simulink model "View_Speed"  (R2024b)
settings: Solver=FixedStepDiscrete  StartTime=0.0  StopTime=10.0  FixedStep=0.1  RelTol=1e-3  EnableMultiTasking=on
values from neighbouring files (symbols this model uses):
  C_BLANK = mpt.Parameter    [View_Speed_dd.m]
  C_CANADA = mpt.Parameter    [View_Speed_dd.m]
  C_DEFAULT_TOLER_A_VALUE = mpt.Parameter    [View_Speed_dd.m]
  C_DEFAULT_TOLER_B_VALUE = mpt.Parameter    [View_Speed_dd.m]
  C_MET_SPD_MAX_VALUE = mpt.Parameter    [View_Speed_dd.m]
  C_MET_SPD_MIN_THRESHOLD = mpt.Parameter    [View_Speed_dd.m]
  C_MEXICO = mpt.Parameter    [View_Speed_dd.m]
  C_SPEED_1KMPH = mpt.Parameter    [View_Speed_dd.m]
  C_SPEED_2KMPH = mpt.Parameter    [View_Speed_dd.m]
  C_SPEED_ZERO = mpt.Parameter    [View_Speed_dd.m]
  C_USA = mpt.Parameter    [View_Speed_dd.m]
  cFACTOR = mpt.Parameter    [View_Speed_dd.m]
  cOFFSET = mpt.Parameter    [View_Speed_dd.m]
  eTOLER_AOut = mpt.Parameter    [View_Speed_dd.m]
  eTOLER_BOut = mpt.Parameter    [View_Speed_dd.m]
  IGN_TRAN_TIMER_MS = mpt.Parameter    [View_Speed_dd.m]
  RESOLUTION_100 = mpt.Parameter    [View_Speed_dd.m]
  RTE_E_MAX_AGE_EXCEEDED = mpt.Parameter    [View_Speed_rte_types.m]
  RTE_E_NEVER_RECEIVED = mpt.Parameter    [View_Speed_rte_types.m]
  VAL_ONE = mpt.Parameter    [View_Speed_dd.m]
  View_Speed_cTaskPeriod = mpt.Parameter    [View_Speed_rte_types.m]
undefined symbols (not defined in the file or in its folder): Arr_u8_100_type_instance, Arr_u8_1024_type_instance, Arr_u8_10_type_instance, Arr_u8_128_type_instance, Arr_u8_16_type_instance, Arr_u8_17_type_instance, Arr_u8_2048_type_instance, Arr_u8_256_type_instance, Arr_u8_32_type_instance, Arr_u8_3_type_instance, Arr_u8_46_type_instance, Arr_u8_48_type_instance, Arr_u8_61_type_instance, Arr_u8_64_type_instance, Arr_u8_8_type_instance, Arr_u8_9_type_instance, CLUSTER_INACTIVE, eMET_SPDOut, eSP_ADR, eSP_CANADA, eSP_ECE, eSP_EUROPE, eSP_KOREA_FMVSS, eSP_KOREA_UN_R, eSP_MEXICO_FMVSS, eSP_MEXICO_UN_R, eSP_UK, eSP_USA, eVehicleSpeedABSIn, IgnOff, IgnOn, pJustRcvdStatus, RxCan_SignalClearJustRcvdStatus, RxCan_SignalGetJustRcvdStatus, RxCan_SignalInvalidProcessingControl, RxCan_SignalMissingProcessingControl, RxCan_SignalNRProcessingControl, SignalId, Status, tRxSignalId_type_instance, tRxSignalJustRcvdStatus_type_instance, tRxSignalStatus_type_instance, tTxSigConfirmStatus_type_instance, tTxSignalId_type_instance, TxCan_ClearCanSignalTxConfirmation
libraries: simulink x8
(part 1 of 2)
settings Model: Creator=AELANGO6  LastModifiedBy=AELANGO6
settings DataIOCC: SaveOutput=off
settings OptimizationCC: DefaultParameterBehavior=Inlined  EnhancedBackFolding=on  PassReuseOutputArgsAs=Individual arguments  ZeroExternalMemoryAtStartup=off  ZeroInternalMemoryAtStartup=off  MaxStackSize=750  OptimizeBlockOrder=speed  DifferentSizesBufferReuse=on  OptimizationCustomize=off  EfficientTunableParamExpr=on
settings DebuggingCC: ParameterTunabilityLossMsg=error
settings SFSimCC: MATLABDynamicMemAlloc=off
settings RTWCC: Description=AUTOSAR  SystemTargetFile=autosar.tlc  GenCodeOnly=on  TemplateMakefile=ert_default_tmf  PortableWordSizes=on  DataTypeReplacement=CDataTypesFixedWidth
settings CodeAppCC: ForceParamTrailComments=on  IgnoreCustomStorageClasses=off  OperatorAnnotations=on  SimulinkDataObjDesc=on  SFDataObjDesc=on  InsertBlockDesc=on
settings STFCustomTargetCC: TargetLangStandard=C99 (ISO)  MultiwordLength=256  ParMdlRefBuildCompliant=on  CompOptLevelCompliant=on  IncludeMdlTerminateFcn=off  CombineOutputUpdateFcns=on  SuppressErrorStatus=on  ERTCustomFileBanners=on  SupportNonFinite=off  SupportComplex=off  SupportContinuousTime=off  SupportNonInlinedSFcns=off  RemoveResetFunc=on  ParenthesesLevel=Maximum  CastingMode=Standards  MATLABClassNameForMDSCustomization=Simulink.SoftwareTarget.ERTCustomization  AutosarCompliant=on  UseToolchainInfoCompliant=on  LookupTableObjectStructAxisOrder=2,1,3,4,...  LUTObjectStructOrderEvenSpacing=Size,Table,Breakpoints  SystemTargetFile=autosar.tlc
settings ERTTargetCC: TargetLangStandard=C99 (ISO)  ConcurrentExecutionCompliant=off  IncludeMdlTerminateFcn=off  SuppressErrorStatus=on  SupportNonFinite=off  SupportComplex=off  ParenthesesLevel=Maximum  CastingMode=Standards  ModelStepFunctionPrototypeControlCompliant=off  CPPClassGenCompliant=off  AutosarCompliant=on  LookupTableObjectStructAxisOrder=2,1,3,4,...  LUTObjectStructOrderEvenSpacing=Size,Table,Breakpoints  ERTCustomFileTemplate=example_file_process.tlc  ERTFilePackagingFormat=CompactWithDataFile  BooleanTrueId=TRUE  BooleanFalseId=FALSE

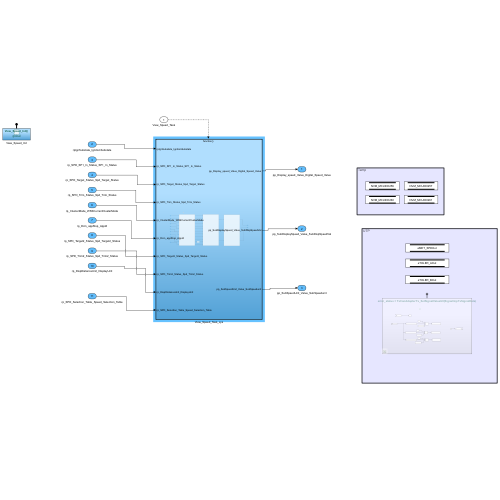
[thumbnail: Simulink's stored preview of the top-level diagram]
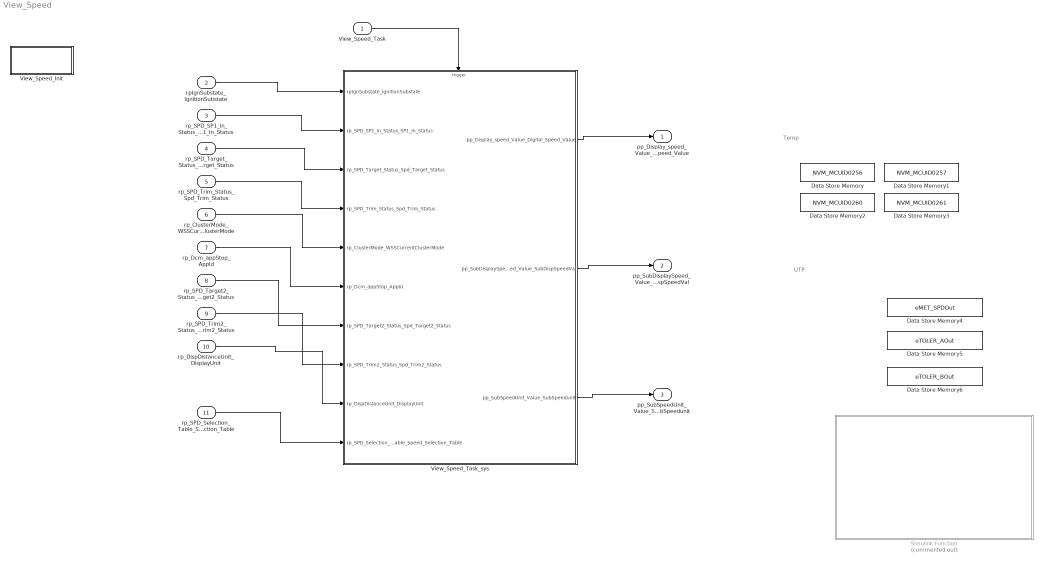
== system View_Speed ==
  note: UTP
  note: Temp
  View_Speed_Task : Inport  SampleTime=0.1  OutputFunctionCall=on
  rpIgnSubstate_IgnitionSubstate : Inport  Port=2  OutDataTypeStr=IgntionSubstateType  PortDimensions=1
  rp_SPD_SP1_In_Status_SP1_In_Status : Inport  Port=3  OutDataTypeStr=uint16  PortDimensions=1
  rp_SPD_Target_Status_Spd_Target_Status : Inport  Port=4  OutDataTypeStr=uint16  PortDimensions=1
  rp_SPD_Trim_Status_Spd_Trim_Status : Inport  Port=5  OutDataTypeStr=uint16  PortDimensions=1
  rp_ClusterMode_WSSCurrentClusterMode : Inport  Port=6  OutDataTypeStr=ClusterModes  PortDimensions=1
  rp_Dcm_appStop_AppId : Inport  Port=7  OutDataTypeStr=IOCtrl_Type  PortDimensions=1
  rp_SPD_Target2_Status_Spd_Target2_Status : Inport  Port=8  OutDataTypeStr=uint16  PortDimensions=1
  rp_SPD_Trim2_Status_Spd_Trim2_Status : Inport  Port=9  OutDataTypeStr=uint16  PortDimensions=1
  rp_DispDistanceUnit_DisplayUnit : Inport  Port=10  OutDataTypeStr=uint8  PortDimensions=1
  rp_SPD_Selection_Table_Speed_Selection_Table : Inport  Port=11  OutDataTypeStr=uint8  PortDimensions=1
  Data Store Memory : DataStoreMemory  DataStoreName=NVM_MCUID0256  ReadBeforeWriteMsg=warning  WriteAfterWriteMsg=warning  WriteAfterReadMsg=warning  InitialValue=C_MCUID0256_VALUE  ShowAdditionalParam=off  OutDataTypeStr=uint16
  Data Store Memory1 : DataStoreMemory  DataStoreName=NVM_MCUID0257  ReadBeforeWriteMsg=warning  WriteAfterWriteMsg=warning  WriteAfterReadMsg=warning  InitialValue=C_MCUID0257_VALUE  ShowAdditionalParam=off  OutDataTypeStr=uint8
  Data Store Memory2 : DataStoreMemory  DataStoreName=NVM_MCUID0260  ReadBeforeWriteMsg=warning  WriteAfterWriteMsg=warning  WriteAfterReadMsg=warning  InitialValue=C_MCUID0260_VALUE  ShowAdditionalParam=off  OutDataTypeStr=uint16
  Data Store Memory3 : DataStoreMemory  DataStoreName=NVM_MCUID0261  ReadBeforeWriteMsg=warning  WriteAfterWriteMsg=warning  WriteAfterReadMsg=warning  InitialValue=C_MCUID0261_VALUE  ShowAdditionalParam=off  OutDataTypeStr=uint8
  Data Store Memory4 : DataStoreMemory  DataStoreName=eMET_SPDOut  ReadBeforeWriteMsg=warning  WriteAfterWriteMsg=warning  WriteAfterReadMsg=warning  ShowAdditionalParam=off  OutDataTypeStr=uint16
  Data Store Memory5 : DataStoreMemory  DataStoreName=eTOLER_AOut  ReadBeforeWriteMsg=warning  WriteAfterWriteMsg=warning  WriteAfterReadMsg=warning  ShowAdditionalParam=off  OutDataTypeStr=uint16
  Data Store Memory6 : DataStoreMemory  DataStoreName=eTOLER_BOut  ReadBeforeWriteMsg=warning  WriteAfterWriteMsg=warning  WriteAfterReadMsg=warning  ShowAdditionalParam=off  OutDataTypeStr=uint16
  Simulink Function : Subsystem  Commented=on  TreatAsAtomicUnit=on
  View_Speed_Init : Subsystem  TreatAsAtomicUnit=on
  View_Speed_Task_sys : Subsystem  TreatAsAtomicUnit=on
  pp_Display_speed_Value_Digital_Speed_Value : Outport  OutDataTypeStr=uint16
  pp_SubDisplaySpeed_Value_SubDispSpeedVal : Outport  Port=2  OutDataTypeStr=uint16
  pp_SubSpeedUnit_Value_SubSpeedunit : Outport  Port=3  OutDataTypeStr=uint8
  wires:
  View_Speed_Task/1 -> View_Speed_Task_sys/Trigger
  rp_SPD_Target2_Status_Spd_Target2_Status/1 -> View_Speed_Task_sys/7(rp_SPD_Target2_Status_Spd_Target2_Status)
  rpIgnSubstate_IgnitionSubstate/1 -> View_Speed_Task_sys/1(rpIgnSubstate_IgnitionSubstate)
  rp_SPD_SP1_In_Status_SP1_In_Status/1 -> View_Speed_Task_sys/2(rp_SPD_SP1_In_Status_SP1_In_Status)
  rp_SPD_Trim_Status_Spd_Trim_Status/1 -> View_Speed_Task_sys/4(rp_SPD_Trim_Status_Spd_Trim_Status)
  rp_SPD_Target_Status_Spd_Target_Status/1 -> View_Speed_Task_sys/3(rp_SPD_Target_Status_Spd_Target_Status)
  rp_Dcm_appStop_AppId/1 -> View_Speed_Task_sys/6(rp_Dcm_appStop_AppId)
  rp_ClusterMode_WSSCurrentClusterMode/1 -> View_Speed_Task_sys/5(rp_ClusterMode_WSSCurrentClusterMode)
  rp_SPD_Trim2_Status_Spd_Trim2_Status/1 -> View_Speed_Task_sys/8(rp_SPD_Trim2_Status_Spd_Trim2_Status)
  rp_DispDistanceUnit_DisplayUnit/1 -> View_Speed_Task_sys/9(rp_DispDistanceUnit_DisplayUnit)
  View_Speed_Task_sys/2(pp_SubDisplaySpeed_Value_SubDispSpeedVal) -> pp_SubDisplaySpeed_Value_SubDispSpeedVal/1
  rp_SPD_Selection_Table_Speed_Selection_Table/1 -> View_Speed_Task_sys/10(rp_SPD_Selection_Table_Speed_Selection_Table)
  View_Speed_Task_sys/1(pp_Display_speed_Value_Digital_Speed_Value) -> pp_Display_speed_Value_Digital_Speed_Value/1
  View_Speed_Task_sys/3(pp_SubSpeedUnit_Value_SubSpeedunit) -> pp_SubSpeedUnit_Value_SubSpeedunit/1

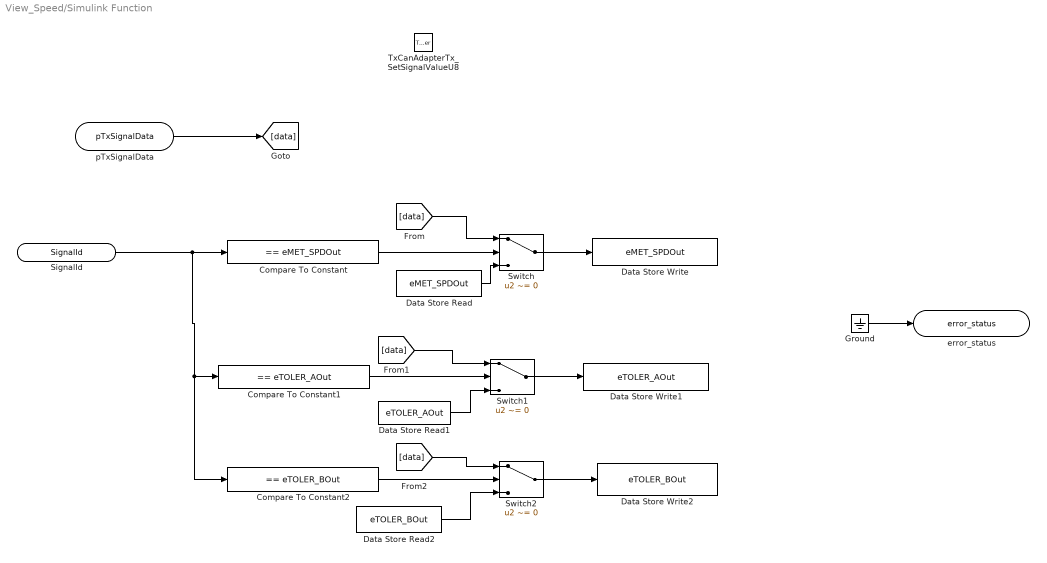
== system View_Speed/Simulink Function ==
  TxCanAdapterTx_SetSignalValueU8 : TriggerPort  TriggerType=function-call  IsSimulinkFunction=on  FunctionName=TxCanAdapterTx_SetSignalValueU8  FunctionVisibility=scoped  VariantControl=(inherit)
  Compare To Constant : simulink/Logic and Bit Operations/Compare To Constant  relop===  const=eMET_SPDOut  OutDataTypeStr=boolean
  Compare To Constant1 : simulink/Logic and Bit Operations/Compare To Constant  relop===  const=eTOLER_AOut  OutDataTypeStr=boolean
  Compare To Constant2 : simulink/Logic and Bit Operations/Compare To Constant  relop===  const=eTOLER_BOut  OutDataTypeStr=boolean
  Data Store Read : DataStoreRead  DataStoreName=eMET_SPDOut  IndexOptions=Index vector (dialog)  Indices=1  OutputSizes=1
  Data Store Read1 : DataStoreRead  DataStoreName=eTOLER_AOut  IndexOptions=Index vector (dialog)  Indices=1  OutputSizes=1
  Data Store Read2 : DataStoreRead  DataStoreName=eTOLER_BOut  IndexOptions=Index vector (dialog)  Indices=1  OutputSizes=1
  Data Store Write : DataStoreWrite  DataStoreName=eMET_SPDOut  IndexOptions=Index vector (dialog)  Indices=1  OutputSizes=1
  Data Store Write1 : DataStoreWrite  DataStoreName=eTOLER_AOut  IndexOptions=Index vector (dialog)  Indices=1  OutputSizes=1
  Data Store Write2 : DataStoreWrite  DataStoreName=eTOLER_BOut  IndexOptions=Index vector (dialog)  Indices=1  OutputSizes=1
  Ground : Ground
  Switch : Switch  Criteria=u2 ~= 0  SaturateOnIntegerOverflow=off  InputSameDT=off
  Switch1 : Switch  Criteria=u2 ~= 0  SaturateOnIntegerOverflow=off  InputSameDT=off
  Switch2 : Switch  Criteria=u2 ~= 0  SaturateOnIntegerOverflow=off  InputSameDT=off
  SignalId : ArgIn  DisableCoverage=on  OutDataTypeStr=uint16  ArgumentName=SignalId
  pTxSignalData : ArgIn  Port=2  OutDataTypeStr=uint8  ArgumentName=pTxSignalData
  error_status : ArgOut  DisableCoverage=on  OutDataTypeStr=uint8  ArgumentName=error_status
  wires:
  SignalId/1 -> Compare To Constant2/1, Compare To Constant1/1, Compare To Constant/1
  Compare To Constant/1 -> Switch/2
  Compare To Constant1/1 -> Switch1/2
  Compare To Constant2/1 -> Switch2/2
  pTxSignalData/1 -> [data]
  [data] -> Switch/1
  [data] -> Switch1/1
  [data] -> Switch2/1
  Switch/1 -> Data Store Write/1
  Switch1/1 -> Data Store Write1/1
  Switch2/1 -> Data Store Write2/1
  Data Store Read/1 -> Switch/3
  Data Store Read1/1 -> Switch1/3
  Data Store Read2/1 -> Switch2/3
  Ground/1 -> error_status/1

== system View_Speed/View_Speed_Init ==
  View_Speed_Init : TriggerPort  TriggerType=function-call  IsSimulinkFunction=on  FunctionName=View_Speed_Init  VariantControl=(inherit)

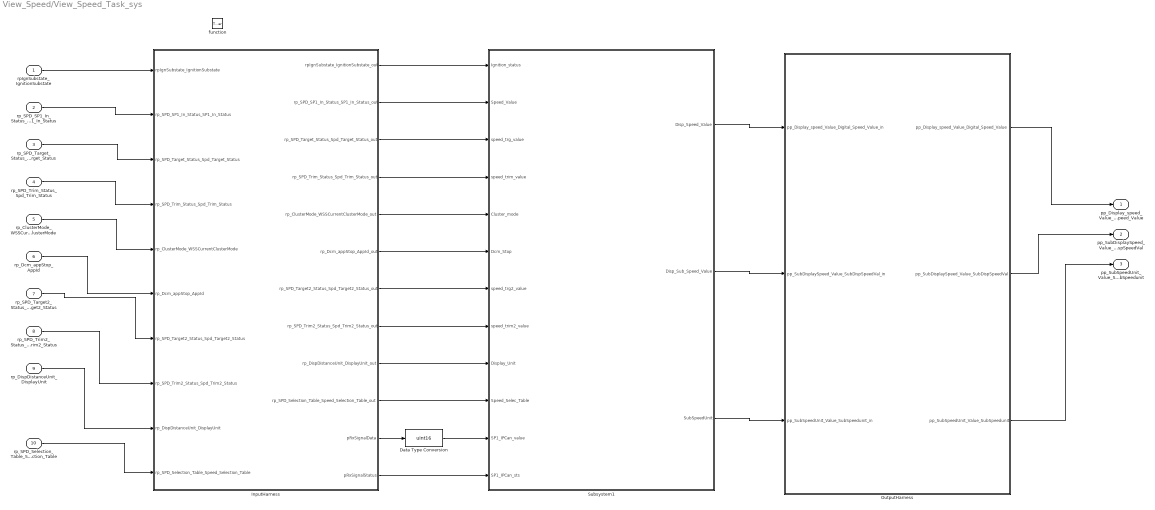
== system View_Speed/View_Speed_Task_sys ==
  rpIgnSubstate_IgnitionSubstate : Inport  OutDataTypeStr=IgntionSubstateType  PortDimensions=1
  rp_SPD_SP1_In_Status_SP1_In_Status : Inport  Port=2  OutDataTypeStr=uint16  PortDimensions=1
  rp_SPD_Target_Status_Spd_Target_Status : Inport  Port=3  OutDataTypeStr=uint16  PortDimensions=1
  rp_SPD_Trim_Status_Spd_Trim_Status : Inport  Port=4  OutDataTypeStr=uint16  PortDimensions=1
  rp_ClusterMode_WSSCurrentClusterMode : Inport  Port=5  OutDataTypeStr=ClusterModes  PortDimensions=1
  rp_Dcm_appStop_AppId : Inport  Port=6  OutDataTypeStr=IOCtrl_Type  PortDimensions=1
  rp_SPD_Target2_Status_Spd_Target2_Status : Inport  Port=7  OutDataTypeStr=uint16  PortDimensions=1
  rp_SPD_Trim2_Status_Spd_Trim2_Status : Inport  Port=8  OutDataTypeStr=uint16  PortDimensions=1
  rp_DispDistanceUnit_DisplayUnit : Inport  Port=9  OutDataTypeStr=uint8  PortDimensions=1
  rp_SPD_Selection_Table_Speed_Selection_Table : Inport  Port=10  OutDataTypeStr=uint8  PortDimensions=1
  function : TriggerPort  TriggerType=function-call  VariantControl=(inherit)  SampleTimeType=periodic  SampleTime=-1
  Data Type Conversion : DataTypeConversion  OutDataTypeStr=uint16  SaturateOnIntegerOverflow=off  RndMeth=Floor
  InputHarness : Subsystem  Variant=on
  OutputHarness : Subsystem  Variant=on
  Subsystem1 : Subsystem
  pp_Display_speed_Value_Digital_Speed_Value : Outport  OutDataTypeStr=uint16  PortDimensions=1
  pp_SubDisplaySpeed_Value_SubDispSpeedVal : Outport  Port=2  OutDataTypeStr=uint16  PortDimensions=1
  pp_SubSpeedUnit_Value_SubSpeedunit : Outport  Port=3  OutDataTypeStr=uint8  PortDimensions=1
  wires:
  rp_SPD_Trim_Status_Spd_Trim_Status/1 -> InputHarness/4(rp_SPD_Trim_Status_Spd_Trim_Status)
  rp_SPD_Target_Status_Spd_Target_Status/1 -> InputHarness/3(rp_SPD_Target_Status_Spd_Target_Status)
  rpIgnSubstate_IgnitionSubstate/1 -> InputHarness/1(rpIgnSubstate_IgnitionSubstate)
  rp_SPD_SP1_In_Status_SP1_In_Status/1 -> InputHarness/2(rp_SPD_SP1_In_Status_SP1_In_Status)
  rp_ClusterMode_WSSCurrentClusterMode/1 -> InputHarness/5(rp_ClusterMode_WSSCurrentClusterMode)
  rp_Dcm_appStop_AppId/1 -> InputHarness/6(rp_Dcm_appStop_AppId)
  rp_SPD_Target2_Status_Spd_Target2_Status/1 -> InputHarness/7(rp_SPD_Target2_Status_Spd_Target2_Status)
  rp_SPD_Trim2_Status_Spd_Trim2_Status/1 -> InputHarness/8(rp_SPD_Trim2_Status_Spd_Trim2_Status)
  rp_DispDistanceUnit_DisplayUnit/1 -> InputHarness/9(rp_DispDistanceUnit_DisplayUnit)
  rp_SPD_Selection_Table_Speed_Selection_Table/1 -> InputHarness/10(rp_SPD_Selection_Table_Speed_Selection_Table)
  OutputHarness/2(pp_SubDisplaySpeed_Value_SubDispSpeedVal) -> pp_SubDisplaySpeed_Value_SubDispSpeedVal/1
  OutputHarness/1(pp_Display_speed_Value_Digital_Speed_Value) -> pp_Display_speed_Value_Digital_Speed_Value/1
  OutputHarness/3(pp_SubSpeedUnit_Value_SubSpeedunit) -> pp_SubSpeedUnit_Value_SubSpeedunit/1
  InputHarness/1(rpIgnSubstate_IgnitionSubstate_out) -> Subsystem1/1(Ignition_status)
  InputHarness/2(rp_SPD_SP1_In_Status_SP1_In_Status_out) -> Subsystem1/2(Speed_Value)
  InputHarness/5(rp_ClusterMode_WSSCurrentClusterMode_out) -> Subsystem1/5(Cluster_mode)
  InputHarness/12(pRxSignalStatus) -> Subsystem1/12(SP1_IPCan_sts)
  InputHarness/10(rp_SPD_Selection_Table_Speed_Selection_Table_out) -> Subsystem1/10(Speed_Selec_Table)
  InputHarness/9(rp_DispDistanceUnit_DisplayUnit_out) -> Subsystem1/9(Display_Unit)
  InputHarness/8(rp_SPD_Trim2_Status_Spd_Trim2_Status_out) -> Subsystem1/8(speed_trim2_value)
  InputHarness/7(rp_SPD_Target2_Status_Spd_Target2_Status_out) -> Subsystem1/7(speed_trg2_value)
  InputHarness/6(rp_Dcm_appStop_AppId_out) -> Subsystem1/6(Dcm_Stop)
  InputHarness/4(rp_SPD_Trim_Status_Spd_Trim_Status_out) -> Subsystem1/4(speed_trim_value)
  InputHarness/3(rp_SPD_Target_Status_Spd_Target_Status_out) -> Subsystem1/3(speed_trg_value)
  Subsystem1/1(Disp_Speed_Value) -> OutputHarness/1(pp_Display_speed_Value_Digital_Speed_Value_in)
  Subsystem1/2(Disp_Sub_Speed_Value) -> OutputHarness/2(pp_SubDisplaySpeed_Value_SubDispSpeedVal_in)
  Subsystem1/3(SubSpeedUnit) -> OutputHarness/3(pp_SubSpeedUnit_Value_SubSpeedunit_in)
  InputHarness/11(pRxSignalData) -> Data Type Conversion/1
  Data Type Conversion/1 -> Subsystem1/11(SP1_IPCan_value)

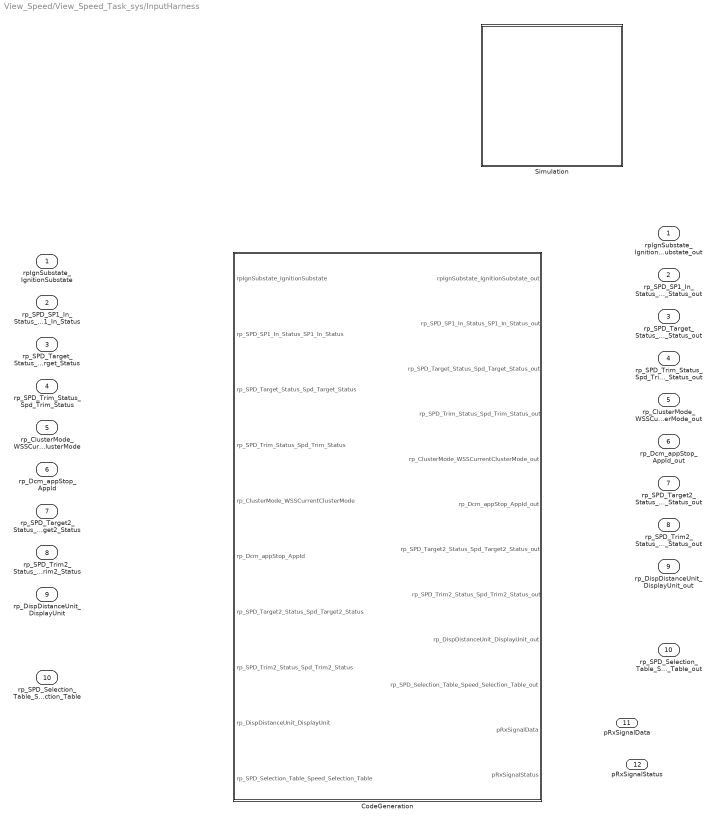
== system View_Speed/View_Speed_Task_sys/InputHarness ==
  rpIgnSubstate_IgnitionSubstate : Inport  OutDataTypeStr=IgntionSubstateType  PortDimensions=1
  rp_SPD_SP1_In_Status_SP1_In_Status : Inport  Port=2  OutDataTypeStr=uint16  PortDimensions=1
  rp_SPD_Target_Status_Spd_Target_Status : Inport  Port=3  OutDataTypeStr=uint16  PortDimensions=1
  rp_SPD_Trim_Status_Spd_Trim_Status : Inport  Port=4  OutDataTypeStr=uint16  PortDimensions=1
  rp_ClusterMode_WSSCurrentClusterMode : Inport  Port=5  OutDataTypeStr=ClusterModes  PortDimensions=1
  rp_Dcm_appStop_AppId : Inport  Port=6  OutDataTypeStr=IOCtrl_Type  PortDimensions=1
  rp_SPD_Target2_Status_Spd_Target2_Status : Inport  Port=7  OutDataTypeStr=uint16  PortDimensions=1
  rp_SPD_Trim2_Status_Spd_Trim2_Status : Inport  Port=8  OutDataTypeStr=uint16  PortDimensions=1
  rp_DispDistanceUnit_DisplayUnit : Inport  Port=9  OutDataTypeStr=uint8  PortDimensions=1
  rp_SPD_Selection_Table_Speed_Selection_Table : Inport  Port=10  OutDataTypeStr=uint8  PortDimensions=1
  CodeGeneration : Subsystem  VariantControl=CODEGENERATION
  Simulation : Subsystem  VariantControl=SIMULATION
  rpIgnSubstate_IgnitionSubstate_out : Outport  OutDataTypeStr=IgntionSubstateType  PortDimensions=1
  rp_SPD_SP1_In_Status_SP1_In_Status_out : Outport  Port=2  OutDataTypeStr=uint16  PortDimensions=1
  rp_SPD_Target_Status_Spd_Target_Status_out : Outport  Port=3  OutDataTypeStr=uint16  PortDimensions=1
  rp_SPD_Trim_Status_Spd_Trim_Status_out : Outport  Port=4  OutDataTypeStr=uint16  PortDimensions=1
  rp_ClusterMode_WSSCurrentClusterMode_out : Outport  Port=5  OutDataTypeStr=ClusterModes  PortDimensions=1
  rp_Dcm_appStop_AppId_out : Outport  Port=6  OutDataTypeStr=IOCtrl_Type  PortDimensions=1
  rp_SPD_Target2_Status_Spd_Target2_Status_out : Outport  Port=7  OutDataTypeStr=uint16  PortDimensions=1
  rp_SPD_Trim2_Status_Spd_Trim2_Status_out : Outport  Port=8  OutDataTypeStr=uint16  PortDimensions=1
  rp_DispDistanceUnit_DisplayUnit_out : Outport  Port=9  OutDataTypeStr=uint8  PortDimensions=1
  rp_SPD_Selection_Table_Speed_Selection_Table_out : Outport  Port=10  OutDataTypeStr=uint8  PortDimensions=1
  pRxSignalData : Outport  Port=11  OutDataTypeStr=uint8  VectorParamsAs1DForOutWhenUnconnected=off
  pRxSignalStatus : Outport  Port=12  OutDataTypeStr=uint8  VectorParamsAs1DForOutWhenUnconnected=off

== system View_Speed/View_Speed_Task_sys/OutputHarness ==
  pp_Display_speed_Value_Digital_Speed_Value_in : Inport  OutDataTypeStr=uint16  PortDimensions=1
  pp_SubDisplaySpeed_Value_SubDispSpeedVal_in : Inport  Port=2  OutDataTypeStr=uint16  PortDimensions=1
  pp_SubSpeedUnit_Value_SubSpeedunit_in : Inport  Port=3  OutDataTypeStr=uint8  PortDimensions=1
  CodeGeneration : Subsystem  VariantControl=CODEGENERATION
  Simulation : Subsystem  VariantControl=SIMULATION
  pp_Display_speed_Value_Digital_Speed_Value : Outport  OutDataTypeStr=uint16  PortDimensions=1
  pp_SubDisplaySpeed_Value_SubDispSpeedVal : Outport  Port=2  OutDataTypeStr=uint16  PortDimensions=1
  pp_SubSpeedUnit_Value_SubSpeedunit : Outport  Port=3  OutDataTypeStr=uint8  PortDimensions=1

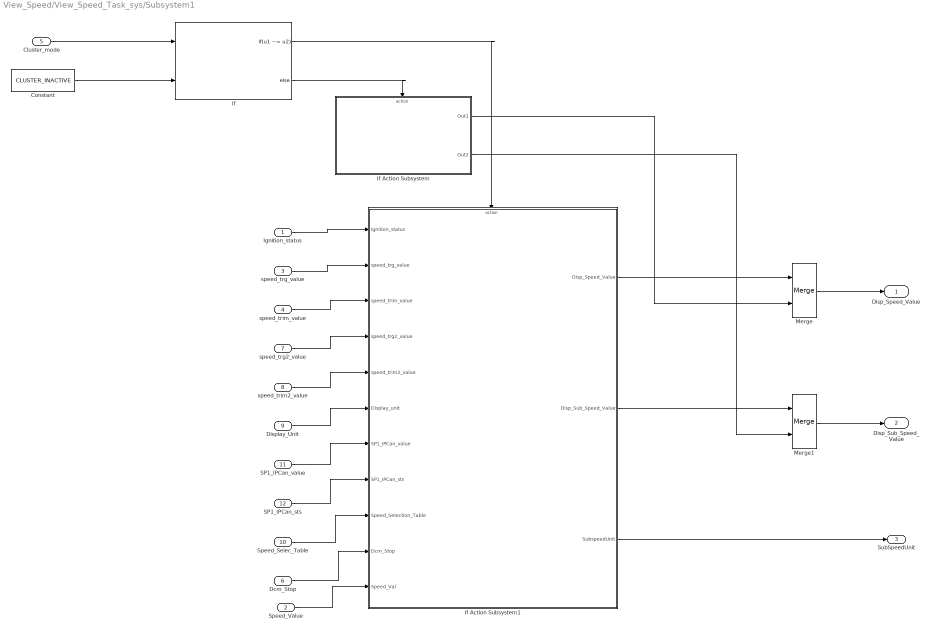
== system View_Speed/View_Speed_Task_sys/Subsystem1 ==
  Ignition_status : Inport
  Speed_Value : Inport  Port=2
  speed_trg_value : Inport  Port=3
  speed_trim_value : Inport  Port=4
  Cluster_mode : Inport  Port=5
  Dcm_Stop : Inport  Port=6
  speed_trg2_value : Inport  Port=7
  speed_trim2_value : Inport  Port=8
  Display_Unit : Inport  Port=9
  Speed_Selec_Table : Inport  Port=10  OutDataTypeStr=uint8
  SP1_IPCan_value : Inport  Port=11  OutDataTypeStr=uint16
  SP1_IPCan_sts : Inport  Port=12  OutDataTypeStr=uint8
  Constant : Constant  Value=CLUSTER_INACTIVE
  If : If  NumInputs=2  IfExpression=u1 ~= u2
  If Action Subsystem : Subsystem  TreatAsAtomicUnit=on
  If Action Subsystem1 : Subsystem  TreatAsAtomicUnit=on
  Merge : Merge
  Merge1 : Merge
  Disp_Speed_Value : Outport  VectorParamsAs1DForOutWhenUnconnected=off
  Disp_Sub_Speed_Value : Outport  Port=2  VectorParamsAs1DForOutWhenUnconnected=off
  SubSpeedUnit : Outport  Port=3  VectorParamsAs1DForOutWhenUnconnected=off
  wires:
  If/2 -> If Action Subsystem/Action
  Cluster_mode/1 -> If/1
  Constant/1 -> If/2
  If/1 -> If Action Subsystem1/Action
  Ignition_status/1 -> If Action Subsystem1/1(Ignition_status)
  speed_trg_value/1 -> If Action Subsystem1/2(speed_trg_value)
  speed_trim_value/1 -> If Action Subsystem1/3(speed_trim_value)
  Dcm_Stop/1 -> If Action Subsystem1/10(Dcm_Stop)
  speed_trim2_value/1 -> If Action Subsystem1/5(speed_trim2_value)
  speed_trg2_value/1 -> If Action Subsystem1/4(speed_trg2_value)
  SP1_IPCan_sts/1 -> If Action Subsystem1/8(SP1_IPCan_sts)
  SP1_IPCan_value/1 -> If Action Subsystem1/7(SP1_IPCan_value)
  Speed_Selec_Table/1 -> If Action Subsystem1/9(Speed_Selection_Table)
  If Action Subsystem1/1(Disp_Speed_Value) -> Merge/1
  If Action Subsystem/1(Out1) -> Merge/2
  If Action Subsystem1/2(Disp_Sub_Speed_Value) -> Merge1/1
  If Action Subsystem/2(Out2) -> Merge1/2
  Merge/1 -> Disp_Speed_Value/1
  Merge1/1 -> Disp_Sub_Speed_Value/1
  Display_Unit/1 -> If Action Subsystem1/6(Display_unit)
  If Action Subsystem1/3(SubspeedUnit) -> SubSpeedUnit/1
  Speed_Value/1 -> If Action Subsystem1/11(Speed_Val)

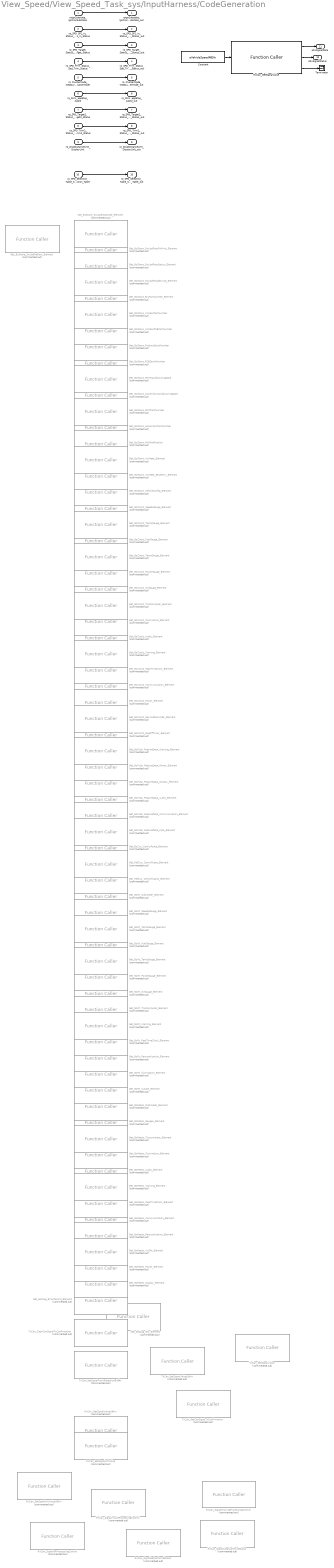
== system View_Speed/View_Speed_Task_sys/InputHarness/CodeGeneration ==
  rpIgnSubstate_IgnitionSubstate : Inport  OutDataTypeStr=IgntionSubstateType  PortDimensions=1
  rp_SPD_SP1_In_Status_SP1_In_Status : Inport  Port=2  OutDataTypeStr=uint16  PortDimensions=1
  rp_SPD_Target_Status_Spd_Target_Status : Inport  Port=3  OutDataTypeStr=uint16  PortDimensions=1
  rp_SPD_Trim_Status_Spd_Trim_Status : Inport  Port=4  OutDataTypeStr=uint16  PortDimensions=1
  rp_ClusterMode_WSSCurrentClusterMode : Inport  Port=5  OutDataTypeStr=ClusterModes  PortDimensions=1
  rp_Dcm_appStop_AppId : Inport  Port=6  OutDataTypeStr=IOCtrl_Type  PortDimensions=1
  rp_SPD_Target2_Status_Spd_Target2_Status : Inport  Port=7  OutDataTypeStr=uint16  PortDimensions=1
  rp_SPD_Trim2_Status_Spd_Trim2_Status : Inport  Port=8  OutDataTypeStr=uint16  PortDimensions=1
  rp_DispDistanceUnit_DisplayUnit : Inport  Port=9  OutDataTypeStr=uint8  PortDimensions=1
  rp_SPD_Selection_Table_Speed_Selection_Table : Inport  Port=10  OutDataTypeStr=uint8  PortDimensions=1
  Constant : Constant  Value=eVehicleSpeedABSIn
  Get_BsConst_Audio_Element : FunctionCaller  Commented=on  FunctionPrototype=[Ptr,error_status] = Get_BsConst_Audio_Element()  InputArgumentSpecifications=<Enter example>  OutputArgumentSpecifications=Arr_u8_128_type_instance(1) ,uint8(1)
  Get_BsConst_Communication_Element : FunctionCaller  Commented=on  FunctionPrototype=[Ptr,error_status] = Get_BsConst_Communication_Element()  InputArgumentSpecifications=<Enter example>  OutputArgumentSpecifications=Arr_u8_64_type_instance(1) ,uint8(1)
  Get_BsConst_EngOffTimer_Element : FunctionCaller  Commented=on  FunctionPrototype=[Ptr,error_status] = Get_BsConst_EngOffTimer_Element()  InputArgumentSpecifications=<Enter example>  OutputArgumentSpecifications=Arr_u8_32_type_instance(1) ,uint8(1)
  Get_BsConst_FuelGauge_Element : FunctionCaller  Commented=on  FunctionPrototype=[Ptr,error_status] = Get_BsConst_FuelGauge_Element()  InputArgumentSpecifications=<Enter example>  OutputArgumentSpecifications=Arr_u8_128_type_instance(1) ,uint8(1)
  Get_BsConst_Illumination_Element : FunctionCaller  Commented=on  FunctionPrototype=[Ptr,error_status] = Get_BsConst_Illumination_Element()  InputArgumentSpecifications=<Enter example>  OutputArgumentSpecifications=Arr_u8_128_type_instance(1) ,uint8(1)
  Get_BsConst_OilGauge_Element : FunctionCaller  Commented=on  FunctionPrototype=[Ptr,error_status] = Get_BsConst_OilGauge_Element()  InputArgumentSpecifications=<Enter example>  OutputArgumentSpecifications=Arr_u8_64_type_instance(1) ,uint8(1)
  Get_BsConst_PowerGauge_Element : FunctionCaller  Commented=on  FunctionPrototype=[Ptr,error_status] = Get_BsConst_PowerGauge_Element()  InputArgumentSpecifications=<Enter example>  OutputArgumentSpecifications=Arr_u8_64_type_instance(1) ,uint8(1)
  Get_BsConst_Power_Element : FunctionCaller  Commented=on  FunctionPrototype=[Ptr,error_status] = Get_BsConst_Power_Element()  InputArgumentSpecifications=<Enter example>  OutputArgumentSpecifications=Arr_u8_32_type_instance(1) ,uint8(1)
  Get_BsConst_RealTimeClock_Element : FunctionCaller  Commented=on  FunctionPrototype=[Ptr,error_status] = Get_BsConst_RealTimeClock_Element()  InputArgumentSpecifications=<Enter example>  OutputArgumentSpecifications=Arr_u8_48_type_instance(1) ,uint8(1)
  Get_BsConst_ServiceReminder_Element : FunctionCaller  Commented=on  FunctionPrototype=[Ptr,error_status] = Get_BsConst_ServiceReminder_Element()  InputArgumentSpecifications=<Enter example>  OutputArgumentSpecifications=Arr_u8_48_type_instance(1) ,uint8(1)
  Get_BsConst_SpeedoGauge_Element : FunctionCaller  Commented=on  FunctionPrototype=[Ptr,error_status] = Get_BsConst_SpeedoGauge_Element()  InputArgumentSpecifications=<Enter example>  OutputArgumentSpecifications=Arr_u8_64_type_instance(1) ,uint8(1)
  Get_BsConst_TachoGauge_Element : FunctionCaller  Commented=on  FunctionPrototype=[Ptr,error_status] = Get_BsConst_TachoGauge_Element()  InputArgumentSpecifications=<Enter example>  OutputArgumentSpecifications=Arr_u8_64_type_instance(1) ,uint8(1)
  Get_BsConst_TempGauge_Element : FunctionCaller  Commented=on  FunctionPrototype=[Ptr,error_status] = Get_BsConst_TempGauge_Element()  InputArgumentSpecifications=<Enter example>  OutputArgumentSpecifications=Arr_u8_64_type_instance(1) ,uint8(1)
  Get_BsConst_TripComputer_Element : FunctionCaller  Commented=on  FunctionPrototype=[Ptr,error_status] = Get_BsConst_TripComputer_Element()  InputArgumentSpecifications=<Enter example>  OutputArgumentSpecifications=Arr_u8_64_type_instance(1) ,uint8(1)
  Get_BsConst_Warning_Element : FunctionCaller  Commented=on  FunctionPrototype=[Ptr,error_status] = Get_BsConst_Warning_Element()  InputArgumentSpecifications=<Enter example>  OutputArgumentSpecifications=Arr_u8_64_type_instance(1) ,uint8(1)
  Get_BsCys_Certicificate_Element : FunctionCaller  Commented=on  FunctionPrototype=[Ptr,error_status] = Get_BsCys_Certicificate_Element()  InputArgumentSpecifications=<Enter example>  OutputArgumentSpecifications=Arr_u8_64_type_instance(1) ,uint8(1)
  Get_BsDiag_Dtc_Element : FunctionCaller  Commented=on  FunctionPrototype=[Ptr,error_status] = Get_BsDiag_Dtc_Element()  InputArgumentSpecifications=<Enter example>  OutputArgumentSpecifications=Arr_u8_2048_type_instance(1) ,uint8(1)
  Get_BsDiag_ErrorRecord_Element : FunctionCaller  Commented=on  FunctionPrototype=[Ptr,error_status] = Get_BsDiag_ErrorRecord_Element()  InputArgumentSpecifications=<Enter example>  OutputArgumentSpecifications=Arr_u8_1024_type_instance(1) ,uint8(1)
  Get_BsFuSa_FeatureData_Audio_Element : FunctionCaller  Commented=on  FunctionPrototype=[Ptr,error_status] = Get_BsFuSa_FeatureData_Audio_Element()  InputArgumentSpecifications=<Enter example>  OutputArgumentSpecifications=Arr_u8_8_type_instance(1) ,uint8(1)
  Get_BsFuSa_FeatureData_Communication_Element : FunctionCaller  Commented=on  FunctionPrototype=[Ptr,error_status] = Get_BsFuSa_FeatureData_Communication_Element()  InputArgumentSpecifications=<Enter example>  OutputArgumentSpecifications=Arr_u8_9_type_instance(1) ,uint8(1)
  Get_BsFuSa_FeatureData_Display_Element : FunctionCaller  Commented=on  FunctionPrototype=[Ptr,error_status] = Get_BsFuSa_FeatureData_Display_Element()  InputArgumentSpecifications=<Enter example>  OutputArgumentSpecifications=uint16(1) ,uint8(1)
  Get_BsFuSa_FeatureData_Fota_Element : FunctionCaller  Commented=on  FunctionPrototype=[Ptr,error_status] = Get_BsFuSa_FeatureData_Fota_Element()  InputArgumentSpecifications=<Enter example>  OutputArgumentSpecifications=uint16(1) ,uint8(1)
  Get_BsFuSa_FeatureData_Power_Element : FunctionCaller  Commented=on  FunctionPrototype=[Ptr,error_status] = Get_BsFuSa_FeatureData_Power_Element()  InputArgumentSpecifications=<Enter example>  OutputArgumentSpecifications=Arr_u8_10_type_instance(1) ,uint8(1)
  Get_BsFuSa_FeatureData_Warning_Element : FunctionCaller  Commented=on  FunctionPrototype=[Ptr,error_status] = Get_BsFuSa_FeatureData_Warning_Element()  InputArgumentSpecifications=<Enter example>  OutputArgumentSpecifications=Arr_u8_3_type_instance(1) ,uint8(1)
  Get_BsReten_Audio_Element : FunctionCaller  Commented=on  FunctionPrototype=[Ptr,error_status] = Get_BsReten_Audio_Element()  InputArgumentSpecifications=<Enter example>  OutputArgumentSpecifications=Arr_u8_100_type_instance(1) ,uint8(1)
  Get_BsReten_Communication_Element : FunctionCaller  Commented=on  FunctionPrototype=[Ptr,error_status] = Get_BsReten_Communication_Element()  InputArgumentSpecifications=<Enter example>  OutputArgumentSpecifications=Arr_u8_100_type_instance(1) ,uint8(1)
  Get_BsReten_Display_Element : FunctionCaller  Commented=on  FunctionPrototype=[Ptr,error_status] = Get_BsReten_Display_Element()  InputArgumentSpecifications=<Enter example>  OutputArgumentSpecifications=Arr_u8_100_type_instance(1) ,uint8(1)
  Get_BsReten_Gauges_Element : FunctionCaller  Commented=on  FunctionPrototype=[Ptr,error_status] = Get_BsReten_Gauges_Element()  InputArgumentSpecifications=<Enter example>  OutputArgumentSpecifications=Arr_u8_100_type_instance(1) ,uint8(1)
  Get_BsReten_Illumination_Element : FunctionCaller  Commented=on  FunctionPrototype=[Ptr,error_status] = Get_BsReten_Illumination_Element()  InputArgumentSpecifications=<Enter example>  OutputArgumentSpecifications=Arr_u8_100_type_instance(1) ,uint8(1)
  Get_BsReten_Odometer_Element : FunctionCaller  Commented=on  FunctionPrototype=[Ptr,error_status] = Get_BsReten_Odometer_Element()  InputArgumentSpecifications=<Enter example>  OutputArgumentSpecifications=Arr_u8_100_type_instance(1) ,uint8(1)
  Get_BsReten_Personalization_Element : FunctionCaller  Commented=on  FunctionPrototype=[Ptr,error_status] = Get_BsReten_Personalization_Element()  InputArgumentSpecifications=<Enter example>  OutputArgumentSpecifications=Arr_u8_100_type_instance(1) ,uint8(1)
  Get_BsReten_Power_Element : FunctionCaller  Commented=on  FunctionPrototype=[Ptr,error_status] = Get_BsReten_Power_Element()  InputArgumentSpecifications=<Enter example>  OutputArgumentSpecifications=Arr_u8_100_type_instance(1) ,uint8(1)
  Get_BsReten_RealTimeClock_Element : FunctionCaller  Commented=on  FunctionPrototype=[Ptr,error_status] = Get_BsReten_RealTimeClock_Element()  InputArgumentSpecifications=<Enter example>  OutputArgumentSpecifications=Arr_u8_100_type_instance(1) ,uint8(1)
  Get_BsReten_Tripcomputer_Element : FunctionCaller  Commented=on  FunctionPrototype=[Ptr,error_status] = Get_BsReten_Tripcomputer_Element()  InputArgumentSpecifications=<Enter example>  OutputArgumentSpecifications=Arr_u8_100_type_instance(1) ,uint8(1)
  Get_BsReten_VisDlt_Element : FunctionCaller  Commented=on  FunctionPrototype=[Ptr,error_status] = Get_BsReten_VisDlt_Element()  InputArgumentSpecifications=<Enter example>  OutputArgumentSpecifications=Arr_u8_256_type_instance(1) ,uint8(1)
  Get_BsReten_Warning_Element : FunctionCaller  Commented=on  FunctionPrototype=[Ptr,error_status] = Get_BsReten_Warning_Element()  InputArgumentSpecifications=<Enter example>  OutputArgumentSpecifications=Arr_u8_100_type_instance(1) ,uint8(1)
  Get_BsRt_CusDlt_Element : FunctionCaller  Commented=on  FunctionPrototype=[Ptr,error_status] = Get_BsRt_CusDlt_Element()  InputArgumentSpecifications=<Enter example>  OutputArgumentSpecifications=Arr_u8_128_type_instance(1) ,uint8(1)
  Get_BsRt_FuelGauge_Element : FunctionCaller  Commented=on  FunctionPrototype=[Ptr,error_status] = Get_BsRt_FuelGauge_Element()  InputArgumentSpecifications=<Enter example>  OutputArgumentSpecifications=Arr_u8_32_type_instance(1) ,uint8(1)
  Get_BsRt_Illumination_Element : FunctionCaller  Commented=on  FunctionPrototype=[Ptr,error_status] = Get_BsRt_Illumination_Element()  InputArgumentSpecifications=<Enter example>  OutputArgumentSpecifications=Arr_u8_100_type_instance(1) ,uint8(1)
  Get_BsRt_Odometer_Element : FunctionCaller  Commented=on  FunctionPrototype=[Ptr,error_status] = Get_BsRt_Odometer_Element()  InputArgumentSpecifications=<Enter example>  OutputArgumentSpecifications=Arr_u8_128_type_instance(1) ,uint8(1)
  Get_BsRt_OilGauge_Element : FunctionCaller  Commented=on  FunctionPrototype=[Ptr,error_status] = Get_BsRt_OilGauge_Element()  InputArgumentSpecifications=<Enter example>  OutputArgumentSpecifications=Arr_u8_8_type_instance(1) ,uint8(1)
  Get_BsRt_Personalization_Element : FunctionCaller  Commented=on  FunctionPrototype=[Ptr,error_status] = Get_BsRt_Personalization_Element()  InputArgumentSpecifications=<Enter example>  OutputArgumentSpecifications=Arr_u8_128_type_instance(1) ,uint8(1)
  Get_BsRt_PowerGauge_Element : FunctionCaller  Commented=on  FunctionPrototype=[Ptr,error_status] = Get_BsRt_PowerGauge_Element()  InputArgumentSpecifications=<Enter example>  OutputArgumentSpecifications=Arr_u8_32_type_instance(1) ,uint8(1)
  Get_BsRt_RealTimeClock_Element : FunctionCaller  Commented=on  FunctionPrototype=[Ptr,error_status] = Get_BsRt_RealTimeClock_Element()  InputArgumentSpecifications=<Enter example>  OutputArgumentSpecifications=Arr_u8_48_type_instance(1) ,uint8(1)
  Get_BsRt_SpeedoGauge_Element : FunctionCaller  Commented=on  FunctionPrototype=[Ptr,error_status] = Get_BsRt_SpeedoGauge_Element()  InputArgumentSpecifications=<Enter example>  OutputArgumentSpecifications=Arr_u8_8_type_instance(1) ,uint8(1)
  Get_BsRt_TachoGauge_Element : FunctionCaller  Commented=on  FunctionPrototype=[Ptr,error_status] = Get_BsRt_TachoGauge_Element()  InputArgumentSpecifications=<Enter example>  OutputArgumentSpecifications=Arr_u8_16_type_instance(1) ,uint8(1)
  Get_BsRt_TempGauge_Element : FunctionCaller  Commented=on  FunctionPrototype=[Ptr,error_status] = Get_BsRt_TempGauge_Element()  InputArgumentSpecifications=<Enter example>  OutputArgumentSpecifications=Arr_u8_32_type_instance(1) ,uint8(1)
  Get_BsRt_TripComputer_Element : FunctionCaller  Commented=on  FunctionPrototype=[Ptr,error_status] = Get_BsRt_TripComputer_Element()  InputArgumentSpecifications=<Enter example>  OutputArgumentSpecifications=Arr_u8_64_type_instance(1) ,uint8(1)
  Get_BsRt_Warning_Element : FunctionCaller  Commented=on  FunctionPrototype=[Ptr,error_status] = Get_BsRt_Warning_Element()  InputArgumentSpecifications=<Enter example>  OutputArgumentSpecifications=Arr_u8_32_type_instance(1) ,uint8(1)
  Get_BsShare_AssemblyManufacturingDate : FunctionCaller  Commented=on  FunctionPrototype=[Ptr,error_status] = Get_BsShare_AssemblyManufacturingDate()  InputArgumentSpecifications=<Enter example>  OutputArgumentSpecifications=Arr_u8_3_type_instance(1) ,uint8(1)
  Get_BsShare_AssemblyPlantNumber : FunctionCaller  Commented=on  FunctionPrototype=[Ptr,error_status] = Get_BsShare_AssemblyPlantNumber()  InputArgumentSpecifications=<Enter example>  OutputArgumentSpecifications=Arr_u8_3_type_instance(1) ,uint8(1)
  Get_BsShare_EcuPartNumber_Element : FunctionCaller  Commented=on  FunctionPrototype=[Ptr,error_status] = Get_BsShare_EcuPartNumber_Element()  InputArgumentSpecifications=<Enter example>  OutputArgumentSpecifications=Arr_u8_61_type_instance(1) ,uint8(1)
  Get_BsShare_HWModification : FunctionCaller  Commented=on  FunctionPrototype=[Ptr,error_status] = Get_BsShare_HWModification()  InputArgumentSpecifications=<Enter example>  OutputArgumentSpecifications=uint16(1) ,uint8(1)
  Get_BsShare_PCBSerialNumber : FunctionCaller  Commented=on  FunctionPrototype=[Ptr,error_status] = Get_BsShare_PCBSerialNumber()  InputArgumentSpecifications=<Enter example>  OutputArgumentSpecifications=Arr_u8_9_type_instance(1) ,uint8(1)
  Get_BsShare_ProductSerialNumber : FunctionCaller  Commented=on  FunctionPrototype=[Ptr,error_status] = Get_BsShare_ProductSerialNumber()  InputArgumentSpecifications=<Enter example>  OutputArgumentSpecifications=Arr_u8_10_type_instance(1) ,uint8(1)
  Get_BsShare_SMTManufacturingDate : FunctionCaller  Commented=on  FunctionPrototype=[Ptr,error_status] = Get_BsShare_SMTManufacturingDate()  InputArgumentSpecifications=<Enter example>  OutputArgumentSpecifications=Arr_u8_3_type_instance(1) ,uint8(1)
  Get_BsShare_SMTPlantNumber : FunctionCaller  Commented=on  FunctionPrototype=[Ptr,error_status] = Get_BsShare_SMTPlantNumber()  InputArgumentSpecifications=<Enter example>  OutputArgumentSpecifications=Arr_u8_3_type_instance(1) ,uint8(1)
  Get_BsShare_SwUpdFotaFinPrint_Element : FunctionCaller  Commented=on  FunctionPrototype=[Ptr,error_status] = Get_BsShare_SwUpdFotaFinPrint_Element()  InputArgumentSpecifications=<Enter example>  OutputArgumentSpecifications=Arr_u8_32_type_instance(1) ,uint8(1)
  Get_BsShare_SwUpdFotaMode_Element : FunctionCaller  Commented=on  FunctionPrototype=[Ptr,error_status] = Get_BsShare_SwUpdFotaMode_Element()  InputArgumentSpecifications=<Enter example>  OutputArgumentSpecifications=Arr_u8_16_type_instance(1) ,uint8(1)
  Get_BsShare_SwUpdFotaStatus_Element : FunctionCaller  Commented=on  FunctionPrototype=[Ptr,error_status] = Get_BsShare_SwUpdFotaStatus_Element()  InputArgumentSpecifications=<Enter example>  OutputArgumentSpecifications=Arr_u8_48_type_instance(1) ,uint8(1)
  Get_BsShare_SwUpdFotadecrypt_Element : FunctionCaller  Commented=on  FunctionPrototype=[Ptr,error_status] = Get_BsShare_SwUpdFotadecrypt_Element()  InputArgumentSpecifications=<Enter example>  OutputArgumentSpecifications=Arr_u8_64_type_instance(1) ,uint8(1)
  Get_BsShare_SwUpdReflash_Element : FunctionCaller  Commented=on  FunctionPrototype=[Ptr,error_status] = Get_BsShare_SwUpdReflash_Element()  InputArgumentSpecifications=<Enter example>  OutputArgumentSpecifications=Arr_u8_8_type_instance(1) ,uint8(1)
  Get_BsShare_VehicleConfig_Element : FunctionCaller  Commented=on  FunctionPrototype=[Ptr,error_status] = Get_BsShare_VehicleConfig_Element()  InputArgumentSpecifications=<Enter example>  OutputArgumentSpecifications=Arr_u8_256_type_instance(1) ,uint8(1)
  Get_BsShare_VisMeet_EOLEntry_Element : FunctionCaller  Commented=on  FunctionPrototype=[Ptr,error_status] = Get_BsShare_VisMeet_EOLEntry_Element()  InputArgumentSpecifications=<Enter example>  OutputArgumentSpecifications=uint16(1) ,uint8(1)
  Get_BsShare_VisMeet_Element : FunctionCaller  Commented=on  FunctionPrototype=[Ptr,error_status] = Get_BsShare_VisMeet_Element()  InputArgumentSpecifications=<Enter example>  OutputArgumentSpecifications=Arr_u8_46_type_instance(1) ,uint8(1)
  Get_BsShare_VisteonPCBPartNumber : FunctionCaller  Commented=on  FunctionPrototype=[Ptr,error_status] = Get_BsShare_VisteonPCBPartNumber()  InputArgumentSpecifications=<Enter example>  OutputArgumentSpecifications=Arr_u8_17_type_instance(1) ,uint8(1)
  Get_BsShare_VisteonPartNumber : FunctionCaller  Commented=on  FunctionPrototype=[Ptr,error_status] = Get_BsShare_VisteonPartNumber()  InputArgumentSpecifications=<Enter example>  OutputArgumentSpecifications=Arr_u8_17_type_instance(1) ,uint8(1)
  Get_RefCys_Certicificate1_Element : FunctionCaller  Commented=on  FunctionPrototype=[Ptr,error_status] = Get_RefCys_Certicificate1_Element()  InputArgumentSpecifications=<Enter example>  OutputArgumentSpecifications=Arr_u8_64_type_instance(1) ,uint8(1)
  Get_RefCys_Certicificate_Element : FunctionCaller  Commented=on  FunctionPrototype=[Ptr,error_status] = Get_RefCys_Certicificate_Element()  InputArgumentSpecifications=<Enter example>  OutputArgumentSpecifications=Arr_u8_64_type_instance(1) ,uint8(1)
  RxCan_GetSignalValue : FunctionCaller  FunctionPrototype=[pSignalValue,pSignalStatus,error_status] = RxCan_GetSignalValue(SignalId)  InputArgumentSpecifications=tRxSignalId_type_instance(1)  OutputArgumentSpecifications=uint8(1) ,tRxSignalStatus_type_instance(1) ,uint8(1)
  RxCan_GetSignalValueU8Arr : FunctionCaller  Commented=on  FunctionPrototype=[pSignalValue,pSignalStatus,pSignalLength,error_status] = RxCan_GetSignalValueU8Arr(SignalId)  InputArgumentSpecifications=tRxSignalId_type_instance(1)  OutputArgumentSpecifications=uint8(1) ,tRxSignalStatus_type_instance(1) ,uint32(1) ,uint8(1)
  RxCan_SetSignalInitValue : FunctionCaller  Commented=on  FunctionPrototype=[pSignalValue,error_status] = RxCan_SetSignalInitValue(SignalId)  InputArgumentSpecifications=tRxSignalId_type_instance(1)  OutputArgumentSpecifications=uint8(1) ,uint8(1)
  RxCan_SetSignalInitValueU8Arr : FunctionCaller  Commented=on  FunctionPrototype=[pSignaValue,pSignalLength,error_status] = RxCan_SetSignalInitValueU8Arr(SignalId)  InputArgumentSpecifications=tRxSignalId_type_instance(1)  OutputArgumentSpecifications=uint8(1) ,uint32(1) ,uint8(1)
  RxCan_SignalClearJustRcvdStatus : FunctionCaller  Commented=on  FunctionPrototype=RxCan_SignalClearJustRcvdStatus(SignalId)  InputArgumentSpecifications=tRxSignalId_type_instance(1)  OutputArgumentSpecifications=<Enter example>
  RxCan_SignalGetJustRcvdStatus : FunctionCaller  Commented=on  FunctionPrototype=RxCan_SignalGetJustRcvdStatus(SignalId,pJustRcvdStatus)  InputArgumentSpecifications=tRxSignalId_type_instance(1) ,tRxSignalJustRcvdStatus_type_instance(1)  OutputArgumentSpecifications=<Enter example>
  RxCan_SignalInvalidProcessingControl : FunctionCaller  Commented=on  FunctionPrototype=RxCan_SignalInvalidProcessingControl(SignalId,Status)  InputArgumentSpecifications=tRxSignalId_type_instance(1) ,boolean(1)  OutputArgumentSpecifications=<Enter example>
  RxCan_SignalMissingProcessingControl : FunctionCaller  Commented=on  FunctionPrototype=RxCan_SignalMissingProcessingControl(SignalId,Status)  InputArgumentSpecifications=tRxSignalId_type_instance(1) ,boolean(1)  OutputArgumentSpecifications=<Enter example>
  RxCan_SignalNRProcessingControl : FunctionCaller  Commented=on  FunctionPrototype=RxCan_SignalNRProcessingControl(SignalId,Status)  InputArgumentSpecifications=tRxSignalId_type_instance(1) ,boolean(1)  OutputArgumentSpecifications=<Enter example>
  Terminator : Terminator
  TxCan_ClearCanSignalTxConfirmation : FunctionCaller  Commented=on  FunctionPrototype=TxCan_ClearCanSignalTxConfirmation(SignalId)  InputArgumentSpecifications=tTxSignalId_type_instance(1)  OutputArgumentSpecifications=<Enter example>
  TxCan_GetCanSignalTxConfirmation : FunctionCaller  Commented=on  FunctionPrototype=pStatus = TxCan_GetCanSignalTxConfirmation(SignalId)  InputArgumentSpecifications=tTxSignalId_type_instance(1)  OutputArgumentSpecifications=tTxSigConfirmStatus_type_instance(1)
  TxCan_SetSignalFromRetentionBuffer : FunctionCaller  Commented=on  FunctionPrototype=error_status = TxCan_SetSignalFromRetentionBuffer(SignalId)  InputArgumentSpecifications=tTxSignalId_type_instance(1)  OutputArgumentSpecifications=uint8(1)
  TxCan_SetSignalValue : FunctionCaller  Commented=on  FunctionPrototype=error_status = TxCan_SetSignalValue(SignalId,pTxSignalData)  InputArgumentSpecifications=tTxSignalId_type_instance(1) ,uint8(1)  OutputArgumentSpecifications=uint8(1)
  TxCan_SetSignalValueU8Arr : FunctionCaller  Commented=on  FunctionPrototype=error_status = TxCan_SetSignalValueU8Arr(SignalId,pTxSignalData,SignalLength)  InputArgumentSpecifications=tTxSignalId_type_instance(1) ,uint8(1) ,uint32(1)  OutputArgumentSpecifications=uint8(1)
  rpIgnSubstate_IgnitionSubstate_out : Outport  OutDataTypeStr=IgntionSubstateType  PortDimensions=1
  rp_SPD_SP1_In_Status_SP1_In_Status_out : Outport  Port=2  OutDataTypeStr=uint16  PortDimensions=1
  rp_SPD_Target_Status_Spd_Target_Status_out : Outport  Port=3  OutDataTypeStr=uint16  PortDimensions=1
  rp_SPD_Trim_Status_Spd_Trim_Status_out : Outport  Port=4  OutDataTypeStr=uint16  PortDimensions=1
  rp_ClusterMode_WSSCurrentClusterMode_out : Outport  Port=5  OutDataTypeStr=ClusterModes  PortDimensions=1
  rp_Dcm_appStop_AppId_out : Outport  Port=6  OutDataTypeStr=IOCtrl_Type  PortDimensions=1
  rp_SPD_Target2_Status_Spd_Target2_Status_out : Outport  Port=7  OutDataTypeStr=uint16  PortDimensions=1
  rp_SPD_Trim2_Status_Spd_Trim2_Status_out : Outport  Port=8  OutDataTypeStr=uint16  PortDimensions=1
  rp_DispDistanceUnit_DisplayUnit_out : Outport  Port=9  OutDataTypeStr=uint8  PortDimensions=1
  rp_SPD_Selection_Table_Speed_Selection_Table_out : Outport  Port=10  OutDataTypeStr=uint8  PortDimensions=1
  pRxSignalData : Outport  Port=11  OutDataTypeStr=uint8  VectorParamsAs1DForOutWhenUnconnected=off
  pRxSignalStatus : Outport  Port=12  OutDataTypeStr=uint8  VectorParamsAs1DForOutWhenUnconnected=off
  wires:
  rpIgnSubstate_IgnitionSubstate/1 -> rpIgnSubstate_IgnitionSubstate_out/1
  rp_SPD_SP1_In_Status_SP1_In_Status/1 -> rp_SPD_SP1_In_Status_SP1_In_Status_out/1
  rp_SPD_Target_Status_Spd_Target_Status/1 -> rp_SPD_Target_Status_Spd_Target_Status_out/1
  rp_SPD_Trim_Status_Spd_Trim_Status/1 -> rp_SPD_Trim_Status_Spd_Trim_Status_out/1
  rp_ClusterMode_WSSCurrentClusterMode/1 -> rp_ClusterMode_WSSCurrentClusterMode_out/1
  rp_Dcm_appStop_AppId/1 -> rp_Dcm_appStop_AppId_out/1
  rp_SPD_Target2_Status_Spd_Target2_Status/1 -> rp_SPD_Target2_Status_Spd_Target2_Status_out/1
  rp_SPD_Trim2_Status_Spd_Trim2_Status/1 -> rp_SPD_Trim2_Status_Spd_Trim2_Status_out/1
  rp_DispDistanceUnit_DisplayUnit/1 -> rp_DispDistanceUnit_DisplayUnit_out/1
  rp_SPD_Selection_Table_Speed_Selection_Table/1 -> rp_SPD_Selection_Table_Speed_Selection_Table_out/1
  RxCan_GetSignalValue/1 -> pRxSignalData/1
  RxCan_GetSignalValue/2 -> pRxSignalStatus/1
  RxCan_GetSignalValue/3 -> Terminator/1
  Constant/1 -> RxCan_GetSignalValue/1

== system View_Speed/View_Speed_Task_sys/InputHarness/Simulation ==

== system View_Speed/View_Speed_Task_sys/OutputHarness/CodeGeneration ==
  pp_Display_speed_Value_Digital_Speed_Value_in : Inport  OutDataTypeStr=uint16  PortDimensions=1
  pp_SubDisplaySpeed_Value_SubDispSpeedVal_in : Inport  Port=2  OutDataTypeStr=uint16  PortDimensions=1
  pp_SubSpeedUnit_Value_SubSpeedunit_in : Inport  Port=3  OutDataTypeStr=uint8  PortDimensions=1
  pp_Display_speed_Value_Digital_Speed_Value : Outport  OutDataTypeStr=uint16  PortDimensions=1
  pp_SubDisplaySpeed_Value_SubDispSpeedVal : Outport  Port=2  OutDataTypeStr=uint16  PortDimensions=1
  pp_SubSpeedUnit_Value_SubSpeedunit : Outport  Port=3  OutDataTypeStr=uint8  PortDimensions=1
  wires:
  pp_Display_speed_Value_Digital_Speed_Value_in/1 -> pp_Display_speed_Value_Digital_Speed_Value/1
  pp_SubDisplaySpeed_Value_SubDispSpeedVal_in/1 -> pp_SubDisplaySpeed_Value_SubDispSpeedVal/1
  pp_SubSpeedUnit_Value_SubSpeedunit_in/1 -> pp_SubSpeedUnit_Value_SubSpeedunit/1

== system View_Speed/View_Speed_Task_sys/OutputHarness/Simulation ==
  pp_Display_speed_Value_Digital_Speed_Value : Outport  OutDataTypeStr=uint16  PortDimensions=1
  pp_SubDisplaySpeed_Value_SubDispSpeedVal : Outport  Port=2  OutDataTypeStr=uint16  PortDimensions=1
  pp_SubSpeedUnit_Value_SubSpeedunit : Outport  Port=3  OutDataTypeStr=uint8  PortDimensions=1

== system View_Speed/View_Speed_Task_sys/Subsystem1/If Action Subsystem ==
  Action Port : ActionPort  ActionPortLabel=else
  Constant : Constant  Value=0  OutDataTypeStr=uint16
  Constant1 : Constant  Value=0  OutDataTypeStr=uint16
  Out1 : Outport  VectorParamsAs1DForOutWhenUnconnected=off
  Out2 : Outport  Port=2  VectorParamsAs1DForOutWhenUnconnected=off
  wires:
  Constant/1 -> Out1/1
  Constant1/1 -> Out2/1
